simulink model "blockdemo"  (Simulink 6.3)
settings: Solver=ode45  StartTime=0.0  StopTime=2e-6  RelTol=1e-3
InitFcn:
  | %% DSPBuilder Start
  | alt_dspbuilder_update_model(bdroot)
  | %% DSPBuilder End
libraries: allblocks_alteradspbuilder2 x26
settings Model: Creator=cpurcell  LastModifiedBy=delphick
settings DebuggingCC: MultiTaskDSMMsg=error

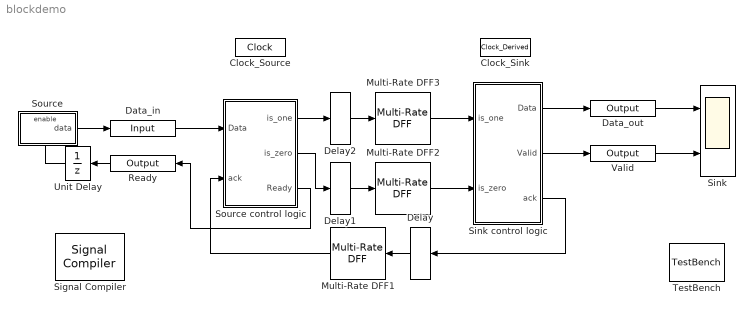
== system blockdemo ==
  Clock_Sink : allblocks_alteradspbuilder2/Clock_Derived  ClockNumerator=1  ClockDenominator=2  SimulationStartCycle=5  PhaseOffset=0  Reset=aclr_sink  Export=off
  Clock_Source : allblocks_alteradspbuilder2/Clock  ClockPeriod=20  ClockPeriodUnit=ns  SampleTime=20e-9  SimulationStartCycle=5  PhaseOffset=0  Reset=aclr_source  Export=off
  Data_in : allblocks_alteradspbuilder2/Input  iofile=C:\workspace_clean\Documentation\DesignExamples\Tutorials\UnitBlocks\RateChange\MultiRateDFF\tb_blockdemo\blockdemo_Data_in.salt  BusType=Single Bit  bwl=8  bwr=0  SpecifyClock=off  PORTTYPE=Input
  Data_out : allblocks_alteradspbuilder2/Output  iofile=C:\workspace_clean\Documentation\DesignExamples\Tutorials\UnitBlocks\RateChange\MultiRateDFF\tb_blockdemo\blockdemo_Data_out.capture  BusType=Single Bit  bwl=8  bwr=0  PORTTYPE=Output
  Delay : allblocks_alteradspbuilder2/Delay  Orientation=left  pipeline=1  ClockPhase=1  use_ena=off  use_sclr=off
  Delay1 : allblocks_alteradspbuilder2/Delay  pipeline=1  ClockPhase=1  use_ena=off  use_sclr=off
  Delay2 : allblocks_alteradspbuilder2/Delay  pipeline=1  ClockPhase=1  use_ena=off  use_sclr=off
  Multi-Rate DFF1 : allblocks_alteradspbuilder2/Multi-Rate DFF  Orientation=left  pipeline=2  UseBaseClock=off  clock=Clock_Source  use_ena=off  use_sclr=off
  Multi-Rate DFF2 : allblocks_alteradspbuilder2/Multi-Rate DFF  pipeline=2  UseBaseClock=off  clock=Clock_Sink  use_ena=off  use_sclr=off
  Multi-Rate DFF3 : allblocks_alteradspbuilder2/Multi-Rate DFF  pipeline=2  UseBaseClock=off  clock=Clock_Sink  use_ena=off  use_sclr=off
  Ready : allblocks_alteradspbuilder2/Output  Orientation=left  iofile=C:\workspace_clean\Documentation\DesignExamples\Tutorials\UnitBlocks\RateChange\MultiRateDFF\tb_blockdemo\blockdemo_Ready.capture  BusType=Single Bit  bwl=8  bwr=0  PORTTYPE=Output
  Signal Compiler : allblocks_alteradspbuilder2/Signal Compiler  DeviceFamily=Stratix IV  DeviceName=AUTO  EnableSignalTap=off  SignalTapDepth=128  UseBoardBlock=off  StpUseDefaultClock=on  StpClock=clock
  Sink : Scope  NumInputPorts=2
      settings: YMin=-0.5~-0.5  YMax=1.5~1.5
  Sink control logic : Subsystem
  Source : Subsystem  TreatAsAtomicUnit=on
  Source control logic : Subsystem
  TestBench : allblocks_alteradspbuilder2/TestBench  enable=on  advancedMode=off  modelSimGui=on  simdatafile=C:\workspace_clean\Documentation\DesignExamples\Tutorials\UnitBlocks\RateChange\MultiRateDFF\tb_blockdemo\blockdemo.simdata.tcl
  Unit Delay : UnitDelay  Orientation=left  SampleTime=-1
  Valid : allblocks_alteradspbuilder2/Output  iofile=C:\workspace_clean\Documentation\DesignExamples\Tutorials\UnitBlocks\RateChange\MultiRateDFF\tb_blockdemo\blockdemo_Valid.capture  BusType=Single Bit  bwl=8  bwr=0  PORTTYPE=Output
  wires:
  Delay1/1 -> Multi-Rate DFF2/1
  Delay/1 -> Multi-Rate DFF1/1
  Delay2/1 -> Multi-Rate DFF3/1
  Multi-Rate DFF2/1 -> Sink control logic/2(is_zero)
  Multi-Rate DFF3/1 -> Sink control logic/1(is_one)
  Data_in/1 -> Source control logic/1(Data)
  Sink control logic/2(Valid) -> Valid/1
  Source/1(data) -> Data_in/1
  Ready/1 -> Unit Delay/1
  Unit Delay/1 -> Source/Enable
  Multi-Rate DFF1/1 -> Source control logic/2(ack)
  Source control logic/1(is_one) -> Delay2/1
  Source control logic/2(is_zero) -> Delay1/1
  Source control logic/3(Ready) -> Ready/1
  Sink control logic/3(ack) -> Delay/1
  Sink control logic/1(Data) -> Data_out/1
  Data_out/1 -> Sink/1
  Valid/1 -> Sink/2

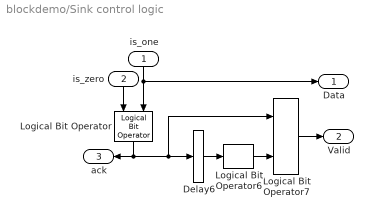
== system blockdemo/Sink control logic ==
  is_one : Inport  Orientation=down
  is_zero : Inport  Orientation=down  Port=2
  Delay6 : allblocks_alteradspbuilder2/Delay  pipeline=1  ClockPhase=1  use_ena=off  use_sclr=off
  Logical Bit Operator : allblocks_alteradspbuilder2/Logical Bit Operator  Orientation=down  LogicalOperator=OR  user_inputs=2
  Logical Bit Operator6 : allblocks_alteradspbuilder2/Logical Bit Operator  LogicalOperator=NOT  user_inputs=2
  Logical Bit Operator7 : allblocks_alteradspbuilder2/Logical Bit Operator  LogicalOperator=AND  user_inputs=2
  Data : Outport
  Valid : Outport  Port=2
  ack : Outport  Orientation=left  Port=3
  wires:
  Logical Bit Operator6/1 -> Logical Bit Operator7/2
  Delay6/1 -> Logical Bit Operator6/1
  Logical Bit Operator/1 -> Delay6/1, Logical Bit Operator7/1, ack/1
  is_one/1 -> Logical Bit Operator/2, Data/1
  is_zero/1 -> Logical Bit Operator/1
  Logical Bit Operator7/1 -> Valid/1

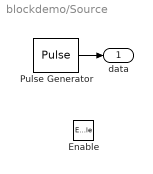
== system blockdemo/Source ==
  Enable : EnablePort
  Pulse Generator : DiscretePulseGenerator  SampleTime=-1
  data : Outport  InitialOutput=0
  wires:
  Pulse Generator/1 -> data/1

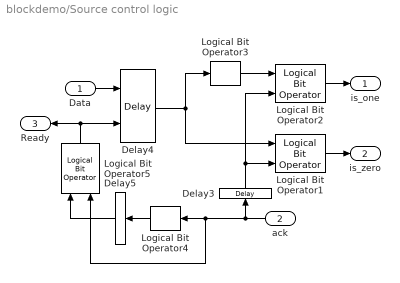
== system blockdemo/Source control logic ==
  Data : Inport
  ack : Inport  Orientation=left  Port=2
  Delay3 : allblocks_alteradspbuilder2/Delay  Orientation=up  pipeline=1  ClockPhase=1  use_ena=off  use_sclr=off
  Delay4 : allblocks_alteradspbuilder2/Delay  pipeline=1  ClockPhase=1  use_ena=on  use_sclr=off
  Delay5 : allblocks_alteradspbuilder2/Delay  Orientation=left  pipeline=1  ClockPhase=1  use_ena=off  use_sclr=off
  Logical Bit Operator1 : allblocks_alteradspbuilder2/Logical Bit Operator  LogicalOperator=NOR  user_inputs=2
  Logical Bit Operator2 : allblocks_alteradspbuilder2/Logical Bit Operator  LogicalOperator=NOR  user_inputs=2
  Logical Bit Operator3 : allblocks_alteradspbuilder2/Logical Bit Operator  LogicalOperator=NOT  user_inputs=2
  Logical Bit Operator4 : allblocks_alteradspbuilder2/Logical Bit Operator  Orientation=left  LogicalOperator=NOT  user_inputs=2
  Logical Bit Operator5 : allblocks_alteradspbuilder2/Logical Bit Operator  Orientation=up  LogicalOperator=NOR  user_inputs=2
  is_one : Outport
  is_zero : Outport  Port=2
  Ready : Outport  Orientation=left  Port=3
  wires:
  Delay3/1 -> Logical Bit Operator1/2, Logical Bit Operator2/2
  ack/1 -> Logical Bit Operator5/2, Logical Bit Operator4/1, Delay3/1
  Logical Bit Operator3/1 -> Logical Bit Operator2/1
  Delay5/1 -> Logical Bit Operator5/1
  Logical Bit Operator5/1 -> Delay4/2, Ready/1
  Logical Bit Operator4/1 -> Delay5/1
  Delay4/1 -> Logical Bit Operator3/1, Logical Bit Operator1/1
  Logical Bit Operator2/1 -> is_one/1
  Data/1 -> Delay4/1
  Logical Bit Operator1/1 -> is_zero/1
